simulink library "pmm"  (R2021b)
settings: Solver=VariableStepAuto  StartTime=0.0  StopTime=10.0  RelTol=1e-3
undefined symbols (not defined in the file or in its folder): APMM_CoolgFanActCurr_X_pct, APMM_EWP1Curr_X_c, APMM_EWP3Curr_X_c, APMM_LVBattChktime_X_enum, APMM_LVBattChrgtime_X_enum, APMM_LVChrgLv_X_mV, ENUM_ANTITHEFT_ALARM, ENUM_ANTITHEFT_ARM, ENUM_ANTITHEFT_DISARM, ENUM_ANTITHEFT_WAIT, ENUM_CHRGPLUGSTA_NONE, ENUM_CRASHSTATE_NOCRASH, ENUM_DCDCFAULTSTA_ANYFAULTLV1, ENUM_DCDCFAULTSTA_ANYFAULTLV2, ENUM_DRIVETRAIN_AWD, ENUM_DRIVETRAIN_FWD, ENUM_DRIVETRAIN_RWD, ENUM_GEARACTUALPOSN_D, ENUM_GEARACTUALPOSN_N, ENUM_GEARACTUALPOSN_R, ENUM_HVBATTREADYPRE_READY, ENUM_OTACHKSTA_NOREQUEST, ENUM_OTACHKSTA_NOTIMEOUT, ENUM_OTACHKSTA_TIMEOUT, ENUM_PDKEYRAWLULOCK_INLOCK, ENUM_PDKEYRAWLULOCK_INUNLOCK, ENUM_PDKEYRAWPS_INPS, ENUM_PDKEYSTA_LOCK, ENUM_PDKEYSTA_PS, ENUM_PDKEYSTA_UNAVALIABLE, ENUM_PDKEYSTA_UNLOCK, ENUM_POWERSTA_OFF, ENUM_POWERSTA_OFFC, ENUM_POWERSTA_STANDBY, ENUM_PWRREQOTA_REQPOWEROFF, ENUM_PWRREQOTA_REQPOWERSTDBY, ENUM_PWRSTASW_READY, FALSE, KPMM_AllDoorClosedHoldTime_s, KPMM_APSAllowThd_pct, KPMM_BattDownFailtime_s, KPMM_BattUpFailtime_s, KPMM_BattUpResetRty_cnt, KPMM_BattUpResetSW_flg, KPMM_BattUpResetTO_s, KPMM_BattUpRstDlyTO_s, KPMM_BrakeSWHoldTime_s, KPMM_ChrgPlugHoldTime_s, KPMM_DCDCDisableFailtime_s, KPMM_DCDCEnableFailtime_s, KPMM_DCDCVSET_V, KPMM_DCDCVSETLVChrg_V, KPMM_DoorSWHoldTime_s, KPMM_DriverSafetyChkFailtime_s, KPMM_DrivetrainSelect_enum_ovrdflg, KPMM_DrivetrainSelect_enum_ovrdval, KPMM_FDADC12VDetAccu_s, KPMM_FDADC12VDetAccuIntval_s, KPMM_FirstLVCheckHoldT_s, KPMM_FrMCUDischrgVolt_V ... (+54)
libraries: simulink x28, hcu_lib x13
(part 2 of 5)

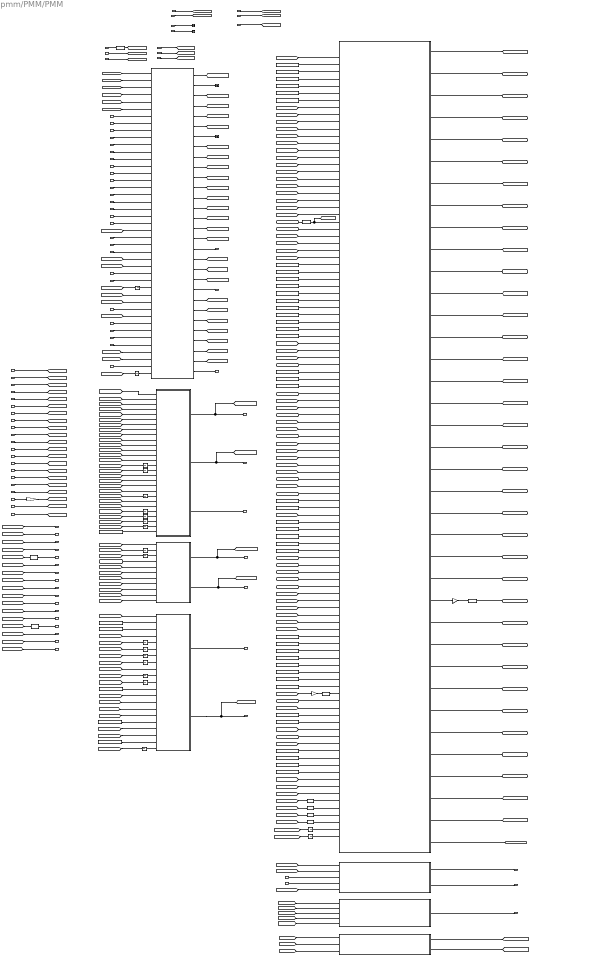
== system pmm/PMM/PMM ==
  note: VPMM_FirstFDADC12VDetAvg_mV
  note: BMS
  note: PEU
  note: 0 = open; 1 = close
  task_time_s : Inport
  VINP_DrDoorSW_flg : Inport  Port=2
  VINP_PsDoorSW_flg : Inport  Port=3
  VINP_RRDoorSW_flg : Inport  Port=4
  VINP_RLDoorSW_flg : Inport  Port=5
  VINP_BrakeSWGPIO_flg : Inport  Port=6
  VINP_SeatSW_flg : Inport  Port=7
  VINP_HoodSW_flg : Inport  Port=8
  VINP_TailgateSW_flg : Inport  Port=9
  VINP_CrashOutputSts_enum : Inport  Port=10
  VINP_VehSpeed_kph : Inport  Port=11
  VINP_IVIPwroffreq_flg : Inport  Port=12
  VINP_IVITriggerreq_flg : Inport  Port=13
  VINP_OFFACMODE_enum : Inport  Port=14
  VINP_AVMOFFRecButt_flg : Inport  Port=15
  VINP_SchedChgwake_flg : Inport  Port=16
  VINP_SchedChgbutt_flg : Inport  Port=17
  VINP_PWCONTINUEUSE_flg : Inport  Port=18
  VINP_DCDCReady4Pre_flg : Inport  Port=19
  VINP_DCDCEnabled_flg : Inport  Port=20
  VINP_OBCEnabled_flg : Inport  Port=21
  VINP_OBCReady4Pre_flg : Inport  Port=22
  VINP_OBCFaultStatus_enum : Inport  Port=23
  VINP_DCDCAuxVolt_V : Inport  Port=24
  VINP_FrMCUDCBusVolt_V : Inport  Port=25
  VINP_FrMCUDischrgSta_flg : Inport  Port=26
  VINP_FrMCUEnaSta_flg : Inport  Port=27
  VINP_FrMCUErr_enum : Inport  Port=28
  VINP_FrMCUReady4Pre_flg : Inport  Port=29
  VINP_FrMCUReady_flg : Inport  Port=30
  VINP_FrMCUTemp_C : Inport  Port=31
  VINP_RrMCUDCBusVolt_V : Inport  Port=32
  VINP_RrMCUDischrgSta_flg : Inport  Port=33
  VINP_RrMCUEnaSta_flg : Inport  Port=34
  VINP_RrMCUErr_enum : Inport  Port=35
  VINP_RrMCUReady4Pre_flg : Inport  Port=36
  VINP_RrMCUReady_flg : Inport  Port=37
  VINP_RrMCUTemp_C : Inport  Port=38
  VINP_HVBattReady4Pre_enum : Inport  Port=39
  VINP_ChrgPlugSta_enum : Inport  Port=40
  VINP_BMSREADY_flg : Inport  Port=41
  VINP_HVILSta_flg : Inport  Port=42
  VINP_HVBContactorSta_flg : Inport  Port=43
  VINP_ExtChrgSta_enum : Inport  Port=44
  VINP_HVBattSOC_pct : Inport  Port=45
  VINP_RrTMSpd_rpm : Inport  Port=46
  VINP_FrTMSpd_rpm : Inport  Port=47
  VINP_OBCPluginSta_flg : Inport  Port=48
  VINP_BMSWarn5_flg : Inport  Port=49
  VINP_BMSWarn6_flg : Inport  Port=50
  VINP_BMSWarn7_flg : Inport  Port=51
  VINP_BMSWarn8_flg : Inport  Port=52
  VINP_HVBPreheatPrecoolSta_enum : Inport  Port=53
  VINP_DCDCFaultSta_enum : Inport  Port=54
  VINP_CANMsgValidBMS2_flg : Inport  Port=55
  VINP_CANMsgValidBMS3_flg : Inport  Port=56
  VINP_FrEDURealTMTq_Nm : Inport  Port=57
  VINP_RrEDURealTMTq_Nm : Inport  Port=58
  VINP_DCDCAuxCur_A : Inport  Port=59
  VINP_V2LSta_enum : Inport  Port=60
  VINP_LVBattDet12V_V : Inport  Port=61
  VINP_PDKeyAreaPS_flg : Inport  Port=62
  VINP_PDKeyAreaLockUnlock_flg : Inport  Port=63
  VINP_PowerOffTSet_cnt : Inport  Port=64
  VINP_RePwrReqTbox_enum : Inport  Port=65
  VTQD_GearActualPosn_enum : Inport  Port=66
  VTQD_PBWLockTO_flg : Inport  Port=67
  VBCM_AntitheftSta_enum : Inport  Port=68
  VINP_AllowMovThd_OTA_enum : Inport  Port=69
  VINP_PwrReq_OTA_enum : Inport  Port=70
  VINP_DrivetrainSelect_enum : Inport  Port=71
  VINP_EvccAplusPwrUpReq_flg : Inport  Port=72
  VDHP_ActAPSPosn_pct : Inport  Port=73
  VDHP_EAPS12RangeSta_enum : Inport  Port=74
  VINP_FDEWP1Cmd_enum : Inport  Port=75
  VINP_FDEWP3Cmd_enum : Inport  Port=76
  VINP_CoolgFanActDuty_pct : Inport  Port=77
  VINP_PowerOffTSetDKC_enum : Inport  Port=78
  VINP_RePwrReqDKCT_enum : Inport  Port=79
  Constant : Constant  Value=KPMM_LVBattChkOKStdT_s
  Constant1 : Constant  Value=KPMM_LVBattThd_V
  Constant10 : Constant  Value=KPMM_OBCDisableFailtime_s
  Constant11 : Constant  Value=KPMM_DriverSafetyChkFailtime_s
  Constant12 : Constant  Value=KPMM_FDADC12VDetAccu_s
  Constant13 : Constant  Value=KPMM_PrechrgChkFailtime_s
  Constant14 : Constant  Value=KPMM_FirstLVCheckHoldT_s
  Constant15 : Constant  Value=KPMM_MLvSafetyFailtime_s
  Constant16 : Constant  Value=KPMM_MCUDisChrgFailtime_s
  Constant17 : Constant  Value=KPMM_DCDCVSET_V
  Constant18 : Constant  Value=KPMM_OFFStaByPassLVBatt_flg
  Constant19 : Constant  Value=KPMM_SilentChrgReq_flg_ovrdflg
  Constant2 : Constant  Value=KPMM_PwrStaStdTO_s
  Constant20 : Constant  Value=KPMM_DCDCEnableFailtime_s
  Constant21 : Constant  Value=KPMM_BattDownFailtime_s
  Constant22 : Constant  Value=KPMM_MCUDisableFailtime_s
  Constant23 : Constant  Value=KPMM_APSAllowThd_pct
  Constant24 : Constant  Value=KPMM_DCDCDisableFailtime_s
  Constant25 : Constant  Value=KPMM_SilentChrgReq_flg_ovrdval
  Constant27 : Constant  Value=KPMM_HVSOCWarnThd_pct
  Constant28 : Constant  Value=KPMM_HVBattSOCPwrDwnThd_pct
  Constant29 : Constant  Value=KPMM_HVSOCWarnThd_pct
  Constant3 : Constant  Value=KPMM_HVBattSOCThd_pct
  Constant30 : Constant  Value=KPMM_OffA2OffTime_s
  Constant31 : Constant  Value=KPMM_PluginVehSpdThd_kph
  Constant32 : Constant  Value=KPMM_LVChrgCurrMthd_flg
  Constant33 : Constant  Value=KPMM_LVChrgHoldT_s
  Constant34 : Constant  Value=KPMM_SysBaseCurr_A
  Constant35 : Constant  Value=KPMM_HVSOCWarnTime_s
  Constant36 : Constant  Value=KPMM_SilentChrgReqTO_s
  Constant37 : Constant  Value=KPMM_PwrStaONTOPop_s
  Constant38 : Constant  Value=KPMM_LVBattChkWakehold_s
  Constant39 : Constant  Value=KPMM_LVBattOFFSlpThd_mV
  Constant4 : Constant  Value=KPMM_HVBSOCOffStaChkFailtime_s
  Constant40 : Constant  Value=KPMM_OFFLVBattChkRetry_cnt
  Constant41 : Constant  Value=KPMM_SysPwrDownDbns_s
  Constant42 : Constant  Value=KPMM_BattUpResetRty_cnt
  Constant43 : Constant  Value=KPMM_BattUpResetSW_flg
  Constant44 : Constant  Value=KPMM_BattUpResetTO_s
  Constant45 : Constant  Value=KPMM_BattUpRstDlyTO_s
  Constant46 : Constant  Value=KPMM_HoodOffChkFailtime_s
  Constant47 : Constant  Value=KPMM_HVBattSOCPwrDwnThd_pct
  Constant5 : Constant  Value=KPMM_HVBSOCOFFCStaChkFailtime_s
  Constant6 : Constant  Value=KPMM_FDADC12VDetAccuIntval_s
  Constant7 : Constant  Value=KPMM_OBCPreChgChkFailtime_s
  Constant8 : Constant  Value=KPMM_SafetyChkFailtime_s
  Constant9 : Constant  Value=KPMM_BattUpFailtime_s  OutDataTypeStr=single
  DCDC output volt setpoint judgment : Subsystem
  Data Type Conversion : DataTypeConversion
  Data Type Conversion1 : DataTypeConversion
  Data Type Conversion2 : DataTypeConversion  OutDataTypeStr=single
  Data Type Conversion3 : DataTypeConversion  OutDataTypeStr=uint8
  Data Type Conversion39 : DataTypeConversion
  Data Type Conversion4 : DataTypeConversion  OutDataTypeStr=single
  Detect Decrease : simulink/Logic and Bit Operations/Detect Decrease  vinit=0.0  OutDataTypeStr=boolean
  Detect Increase : simulink/Logic and Bit Operations/Detect Increase  vinit=0.0  OutDataTypeStr=boolean
  Detect Increase1 : simulink/Logic and Bit Operations/Detect Increase  vinit=0.0  OutDataTypeStr=boolean
  Detect Increase2 : simulink/Logic and Bit Operations/Detect Increase  vinit=0.0  OutDataTypeStr=boolean
  Gain : Gain  Gain=MIN2SEC
  Gain1 : Gain  Gain=1000
  Gain2 : Gain  Gain=0.001
  MCU_EnaReq_Control : Subsystem
  OTA power state constrain : Subsystem
  PMMDataConvert : Subsystem  AncestorBlock=pmm/PMM/PowerModeManagement/PMMDataConvert
  PMM_State_Machine : Stateflow chart  TreatAsAtomicUnit=on
      settings: PortSchema="{\"entries\":[{\"content\":{\"sides\":[{\"content\":{\"connectorIds\":[\"In1\",\"In2\",\"In3\",\"In4\",\"In5\",\"In6\",\"In7\",\"In8\",\"In9\",\"In10\",\"In11\",\"In12\",\"In13\",\"In14\",\"In15\",\"In16\",\"In17\",\"In18\",\"In19\",\"In20\",\"In21\",\"In22\",\"In23\",\"In24\",\"In25\",\"In26\",\"In27\",\"In28\",\"In29\",\"In30\",\"In31\",\"In32\",\"In33\",\"In34\",\"In35\",\"In36\",\"In37\",\"In38\",\"In39\",\"In40\",\"In41\",\"In42\",\"In43\",\"In44\",\"In45\",\"In46\",\"In47\",\"In48\",\"In49\",\"In50\",\"In51\",\"In53\",\"In54\",\"In55\",\"In56\",\"In57\",\"In58\",\"In59\",\"In52\",\"In60\",\"In61\",\"In62\",\"In63\",\"In64\",\"In66\",\"In67\",\"In68\",\"In69\",\"In70\",\"In71\",\"In74\",\"In75\",\"In72\",\"In73\",\"In65\",\"In76\",\"In77\",\"In78\",\"In79\",\"In80\",\"In81\",\"In82\",\"In83\",\"In84\",\"In85\",\"In86\",\"In87\",\"In88\",\"In89\",\"In90\",\"In91\",\"In97\",\"In98\",\"In99\",\"In100\",\"In101\",\"In96\",\"In92\",\"In93\",\"In94\",\"In95\",\"In102\",\"In103\",\"In104\",\"In105\",\"In106\",\"In107\",\"In108\",\"In109\",\"In110\"]},\"type\":\"ConnectorPlacement.EquallySpacedRectSide\",\"uuid\":\"8ab1b0ff-73ed-4b41-8f3f-fcf16c31188d\"},{\"content\":{\"connectorIds\":[\"Out1\",\"Out2\",\"Out3\",\"Out4\",\"Out5\",\"Out6\",\"Out7\",\"Out8\",\"Out9\",\"Out10\",\"Out11\",\"Out12\",\"Out13\",\"Out14\",\"Out17\",\"Out18\",\"Out19\",\"Out20\",\"Out21\",\"Out22\",\"Out23\",\"Out24\",\"Out25\",\"Out26\",\"Out27\",\"Out28\",\"Out29\",\"Out30\",\"Out31\",\"Out32\",\"Out33\",\"Out34\",\"Out35\",\"Out36\",\"Out15\",\"Out16\",\"Out37\"],\"side\":\"RIGHT\"},\"type\":\"ConnectorPlacement.EquallySpacedRectSide\",\"uuid\":\"e75ad163-33ee-46d6-b33a-670f57cb3f5e\"},{\"content\":{\"connectorIds\":[],\"side\":\"TOP\"},\"type\":\"ConnectorPlacement.EquallySpacedRectSide\",\"uuid\":\"84c68278-d5af-48d1-859e-0f05090acbaa\"}]},\"type\":\"ConnectorPlacement.EquallySpacedConnector\",\"uuid\":\"278d3476-0e07-485b-a357-39a0667eafe4\"}],\"packageUris\":[\"http://schema.mathworks.com/mf0/Connector/R2020b\"],\"version\":\"1.0\"}"
  RequirementManagementForPowerDown : Stateflow chart  TreatAsAtomicUnit=on
  RequirementManagementForPowerStateConstrain : Stateflow chart  TreatAsAtomicUnit=on
      settings: PortSchema="{\"entries\":[{\"content\":{\"sides\":[{\"content\":{\"connectorIds\":[\"In1\",\"In2\",\"In11\",\"In3\",\"In4\",\"In5\",\"In6\",\"In7\",\"In8\",\"In9\",\"In10\"]},\"type\":\"ConnectorPlacement.EquallySpacedRectSide\",\"uuid\":\"c4039c9e-34d9-4d76-8a20-7739646b6da6\"},{\"content\":{\"connectorIds\":[\"Out1\",\"Out2\"],\"side\":\"RIGHT\"},\"type\":\"ConnectorPlacement.EquallySpacedRectSide\",\"uuid\":\"63e3e661-9024-478e-a9c0-8e66b2c0118c\"},{\"content\":{\"connectorIds\":[],\"side\":\"TOP\"},\"type\":\"ConnectorPlacement.EquallySpacedRectSide\",\"uuid\":\"6c94eba6-19b8-417a-9a11-c61323531ba8\"}]},\"type\":\"ConnectorPlacement.EquallySpacedConnector\",\"uuid\":\"e4d90d6b-0647-4724-8d20-4a3edeab4c97\"}],\"packageUris\":[\"http://schema.mathworks.com/mf0/Connector/R2020b\"],\"version\":\"1.0\"}"
  RequirementManagementForPowerUp : Stateflow chart  TreatAsAtomicUnit=on
  Terminator{,1..3} (4 alike) : Terminator
  Unit Delay{,1..19} (20 alike) : UnitDelay  SampleTime=-1  HasFrameUpgradeWarning=on
  VPMM_PowerUpState_enum : Outport
  VPMM_PowerDownState_enum : Outport  Port=2
  VPMM_PowerUpFault_enum : Outport  Port=3
  VPMM_PowerDownFault_enum : Outport  Port=4
  VPMM_ActiveDischargeReq_flg : Outport  Port=5
  VPMM_DCDCEnaReq_flg : Outport  Port=6
  VPMM_DCDCVoltSetpoint_V : Outport  Port=7
  VPMM_HVBatCnctReq_flg : Outport  Port=8
  VPMM_HVSysReadyToCharge_enum : Outport  Port=9
  VPMM_PowerSta_enum : Outport  Port=10
  VPMM_LVPwrSta_flg : Outport  Port=11
  VPMM_HVPwrSta_flg : Outport  Port=12
  VPMM_SysPowerMode_enum : Outport  Port=13
  VPMM_FrMCUEnaReq_flg : Outport  Port=14
  VPMM_RrMCUEnaReq_flg : Outport  Port=15
  VPMM_DrivetrainSelect_enum : Outport  Port=16
  VPMM_DrSeatSta_enum : Outport  Port=17
  VPMM_PwrStaSelect_enum : Outport  Port=18
  VPMM_PwrStaConstraint_enum : Outport  Port=19
  VPMM_TCountSta_enum : Outport  Port=20
  VPMM_PwrUpReq_enum : Outport  Port=21
  VPMM_PwrDownReq_enum : Outport  Port=22
  VPMM_LowSOCWarn_enum : Outport  Port=23
  VPMM_ReVehThdChkSta_enum : Outport  Port=24
  VPMM_LVSysErrPwrOutErr_flg : Outport  Port=25
  VPMM_EvccAplusPwrUpReq_flg : Outport  Port=26
  VPMM_PwrStaONTOPopReq_flg : Outport  Port=27
  VPMM_IVIPwrStaONTOPopT_s : Outport  Port=28
  VPMM_LVChrgHoldTtimer_s : Outport  Port=29
  VPMM_LVBattChrgTimeCnt_s : Outport  Port=30
  VPMM_SilentChkAllowSleep_flg : Outport  Port=31
  VPMM_TimerAllowSleep_flg : Outport  Port=32
  VPMM_FDADC12VDetAvg_mV : Outport  Port=33
  VPMM_PMMAllowECUSleep_flg : Outport  Port=34
  VPMM_LVSilentChrgSta_enum : Outport  Port=35
  VPMM_LVSilentChrgReq_flg : Outport  Port=36
  VPMM_LVSilentChrgLv_enum : Outport  Port=37
  VPMM_LVBattChktime_s : Outport  Port=38
  VPMM_SafetyChkMLv_flg : Outport  Port=39
  VPMM_SafetyChkHLv_flg : Outport  Port=40
  VPMM_HVChrgPreActionErrSta_enum : Outport  Port=41
  VPMM_MCUReady_flg : Outport  Port=42
  VPMM_MCUReady4Pre_flg : Outport  Port=43
  VPMM_CtrlFrPwrStbA1P_flg : Outport  Port=44
  VPMM_CtrlFrRC1_flg : Outport  Port=45
  VPMM_CtrlFrBMSCCUCIR_flg : Outport  Port=46
  VPMM_CtrlFrEDUINVERTER_flg : Outport  Port=47
  VPMM_HWResetSta_enum : Outport  Port=48
  VPMM_CtrlDrPwrStbA2_flg : Outport  Port=49
  VPMM_PwrStaTOSta_enum : Outport  Port=50
  VPMM_PMMAllowNMSleep_flg : Outport  Port=51
  VPMM_Sched_ChgTOSta_enum : Outport  Port=52
  VPMM_PwrReq_OTA_enum : Outport  Port=53
  VPMM_OTAPwrReqOFFChkSta_enum : Outport  Port=54
  VPMM_OTAPwrReqStdChkSta_enum : Outport  Port=55
  VPMM_MCUDCBusMaxVolt_V : Outport  Port=56
  wires:
  PMM_State_Machine/16(VPMM_PwrStaTOSta_enum) -> [VPMM_PwrStaTOSta_enum]  "VPMM_PwrStaTOSta_enum"
  PMM_State_Machine/17(VPMM_Sched_ChgTOSta_enum) -> [VPMM_Sched_ChgTOSta_enum]  "VPMM_Sched_ChgTOSta_enum"
  PMM_State_Machine/15(VPMM_LVSilentChrgReq_flg) -> [VPMM_LVSilentChrgReq_flg]  "VPMM_LVSilentChrgReq_flg"
  PMM_State_Machine/18(VPMM_LVSilentChrgReqStd_flg) -> [VPMM_LVSilentChrgReqStd_flg]  "VPMM_LVSilentChrgReqStd_flg"
  VDHP_EAPS12RangeSta_enum/1 -> PMM_State_Machine/65(VDHP_EAPS12RangeSta_enum)
  Constant2/1 -> PMM_State_Machine/64(KPMM_PwrStaStdTO_s)
  Constant/1 -> PMM_State_Machine/63(KPMM_LVBattChkOKStdT_s)
  [VINP_EvccAplusPwrUpReq_flg] -> RequirementManagementForPowerUp/23(VINP_EvccAplusPwrUpReq_flg)
  VINP_EvccAplusPwrUpReq_flg/1 -> [VINP_EvccAplusPwrUpReq_flg]
  [VPMM_LVSilentChrgReqStd_flg] -> Unit Delay8/1
  Unit Delay8/1 -> RequirementManagementForPowerUp/24(VPMM_LVSilentChrgReqStd_flg)
  [VINP_ChrgPlugSta_enum] -> RequirementManagementForPowerUp/22(VINP_ChrgPlugSta_enum)
  [VINP_PwrReq_OTA_enum] -> PMM_State_Machine/61(VINP_PwrReq_OTA_enum)
  Unit Delay7/1 -> RequirementManagementForPowerDown/10(VPMM_Sched_ChgTOSta_enum)
  [VPMM_Sched_ChgTOSta_enum] -> Unit Delay7/1
  [VPMM_PowerUpState_enum] -> Unit Delay1/1
  Unit Delay1/1 -> RequirementManagementForPowerUp/21(VPMM_PowerUpState_enum)
  [task_time_s] -> RequirementManagementForPowerUp/1(task_time_s)
  [VPMM_DrivetrainSelect_enum] -> MCU_EnaReq_Control/5(VPMM_DrivetrainSelect_enum)
  MCU_EnaReq_Control/2(VPMM_RrMCUEnaReq_flg) -> VPMM_RrMCUEnaReq_flg/1  "VPMM_RrMCUEnaReq_flg"
  MCU_EnaReq_Control/1(VPMM_FrMCUEnaReq_flg) -> VPMM_FrMCUEnaReq_flg/1  "VPMM_FrMCUEnaReq_flg"
  Unit Delay6/1 -> PMMDataConvert/31(VPMM_PowerSta_enum)
  Unit Delay5/1 -> RequirementManagementForPowerDown/5(VPMM_PowerSta_enum)
  Unit Delay4/1 -> RequirementManagementForPowerStateConstrain/2(VPMM_PowerSta_enum)
  Unit Delay3/1 -> RequirementManagementForPowerUp/15(VPMM_LVSilentChrgReq_flg)
  [VPMM_AllDoorClosed_flg] -> RequirementManagementForPowerUp/8(VPMM_AllDoorClosed_flg)
  Unit Delay2/1 -> RequirementManagementForPowerDown/7(VPMM_PwrStaTOSta_enum)
  Unit Delay/1 -> RequirementManagementForPowerUp/16(VPMM_PowerSta_enum)
  VINP_CANMsgValidBMS3_flg/1 -> PMM_State_Machine/60(VINP_CANMsgValidBMS3_flg)
  PMM_State_Machine/14(VPMM_LVBattChktime_s) -> VPMM_LVBattChktime_s/1  "VPMM_LVBattChktime_s"
  [VPMM_PwrUpReq_enum] -> PMM_State_Machine/59(VPMM_PwrUpReq_enum)
  [VPMM_PwrStaSelect_enum] -> PMM_State_Machine/58(VPMM_PwrStaSelect_enum)
  [VPMM_PwrStaConstraint_enum] -> PMM_State_Machine/57(VPMM_PwrStaConstraint_enum)
  [VPMM_PwrDownReq_enum] -> PMM_State_Machine/56(VPMM_PwrDownReq_enum)
  VINP_AllowMovThd_OTA_enum/1 -> PMM_State_Machine/55(VINP_AllowMovThd_OTA_enum)
  [VINP_RePwrReqTbox_enum] -> RequirementManagementForPowerDown/9(VINP_RePwrReqTbox_enum)
  [VPMM_TCountSta_enum] -> Unit Delay12/1
  [VPMM_PwrStaTOSta_enum] -> Unit Delay2/1
  [VINP_HVBattSOC_pct] -> RequirementManagementForPowerDown/4(VINP_HVBattSOC_pct)
  [VINP_RePwrReqTbox_enum] -> RequirementManagementForPowerUp/20(VINP_RePwrReqTbox_enum)
  [VINP_RePwrReqDKCT_enum] -> RequirementManagementForPowerUp/19(VINP_RePwrReqDKCT_enum)
  VINP_PowerOffTSetDKC_enum/1 -> [VINP_PowerOffTSetDKC_enum]
  VINP_RePwrReqDKCT_enum/1 -> [VINP_RePwrReqDKCT_enum]
  VINP_RePwrReqTbox_enum/1 -> [VINP_RePwrReqTbox_enum]
  [VINP_PwrReq_OTA_enum] -> RequirementManagementForPowerUp/18(VINP_PwrReq_OTA_enum)
  VINP_PwrReq_OTA_enum/1 -> [VINP_PwrReq_OTA_enum]
  [VTQD_GearActualPosn_enum] -> RequirementManagementForPowerUp/17(VTQD_GearActualPosn_enum)
  [VTQD_GearActualPosn_enum] -> PMM_State_Machine/29(VTQD_GearActualPosn_enum)
  VTQD_GearActualPosn_enum/1 -> [VTQD_GearActualPosn_enum]
  [VPMM_DetectDoorOpened_flg] -> RequirementManagementForPowerUp/14(VPMM_DetectDoorOpened_flg)
  [VPMM_ChrgPlugInRisingEdge_flg] -> RequirementManagementForPowerUp/13(VPMM_ChrgPlugInRisingEdge_flg)
  [VPMM_LVSilentChrgReq_flg] -> Unit Delay3/1
  [VPMM_BrkPedalRisingEdge_flg] -> RequirementManagementForPowerUp/12(VPMM_BrkPedalRisingEdge_flg)
  [VBCM_AntitheftSta_enum] -> RequirementManagementForPowerUp/9(VBCM_AntitheftSta_enum)
  [VINP_HVBattSOC_pct] -> RequirementManagementForPowerUp/3(VINP_HVBattSOC_pct)
  [VINP_HVBattSOC_pct] -> PMM_State_Machine/28(VINP_HVBattSOC_pct)
  VINP_HVBattSOC_pct/1 -> [VINP_HVBattSOC_pct]
  VINP_SchedChgbutt_flg/1 -> PMM_State_Machine/51(VINP_SchedChgbutt_flg)
  [VINP_TailgateSW_flg] -> RequirementManagementForPowerUp/5(VINP_TailgateSW_flg)
  [VINP_HoodSW_flg] -> RequirementManagementForPowerUp/4(VINP_HoodSW_flg)
  [VINP_HoodSW_flg] -> PMM_State_Machine/54(VINP_HoodSW_flg)
  VINP_TailgateSW_flg/1 -> [VINP_TailgateSW_flg]
  VINP_HoodSW_flg/1 -> [VINP_HoodSW_flg]
  [VINP_HVBPreheatPrecoolSta_enum] -> RequirementManagementForPowerUp/2(VINP_HVBPreheatPrecoolSta_enum)
  VINP_HVBPreheatPrecoolSta_enum/1 -> [VINP_HVBPreheatPrecoolSta_enum]
  [VPMM_PwrStaConstraint_enum] -> Unit Delay11/1
  [VPMM_BrkPedalPressed_flg] -> RequirementManagementForPowerUp/11(VPMM_BrkPedalPressed_flg)
  [VPMM_BMSWarm_flg] -> RequirementManagementForPowerUp/10(VPMM_BMSWarn_flg)
  [VPMM_PowerSta_enum] -> Unit Delay/1
  [VPMM_PowerSta_enum] -> Unit Delay5/1
  [VPMM_PowerSta_enum] -> Unit Delay4/1
  [task_time_s] -> RequirementManagementForPowerDown/1(task_time_s)
  [task_time_s] -> RequirementManagementForPowerStateConstrain/1(task_time_s)
  Constant30/1 -> RequirementManagementForPowerDown/3(KPMM_OffA2OffTime_s)
  Constant29/1 -> RequirementManagementForPowerDown/2(KPMM_HVSOCWarnThd_pct)
  [VBCM_AntitheftSta_enum] -> PMMDataConvert/2(VBCM_AntitheftSta_enum)
  VBCM_AntitheftSta_enum/1 -> [VBCM_AntitheftSta_enum]
  [VPMM_MCUDCBusMaxVolt_V] -> PMM_State_Machine/52(VPMM_MCUDCBusMaxVolt_V)
  [VINP_DrDoorSW_flg] -> PMM_State_Machine/53(VINP_DrDoorSW_flg)
  [VPMM_SeatSWRisingEdge_flg] -> PMM_State_Machine/50(VPMM_SeatSWRisingEdge_flg)
  [VPMM_ChrgPlugOutFallingEdge_flg] -> PMM_State_Machine/49(VPMM_ChrgPlugFallingEdge_flg)
  VINP_OBCPluginSta_flg/1 -> PMM_State_Machine/48(VINP_OBCPluginSta_flg)
  Constant18/1 -> PMM_State_Machine/47(KPMM_OFFStaByPassLVBatt_flg)
  Constant25/1 -> PMM_State_Machine/46(KPMM_SilentChrgReq_flg_ovrdval)
  Constant19/1 -> PMM_State_Machine/45(KPMM_SilentChrgReq_flg_ovrdflg)
  VTQD_PBWLockTO_flg/1 -> PMM_State_Machine/44(VTQD_EnterPGearFail_flg)
  [VPMM_AllDoorCloseRisingEdge_flg] -> PMM_State_Machine/43(VPMM_AllDoorCloseRisingEdge_flg)
  [VINP_DCDCEnabled_flg] -> PMM_State_Machine/41(VINP_DCDCEnabled_flg)
  Constant17/1 -> PMM_State_Machine/40(KPMM_DCDCVSET_V)
  Constant16/1 -> PMM_State_Machine/39(KPMM_MCUDisChrgFailtime_s)
  Constant15/1 -> PMM_State_Machine/38(KPMM_MLvSafetyFailtime_s)
  [VPMM_PDKeySta_enum] -> PMM_State_Machine/26(VPMM_PDKeySta_enum)
  Constant13/1 -> PMM_State_Machine/37(KPMM_PrechrgChkFailtime_s)
  [VINP_SeatSW_flg] -> PMM_State_Machine/27(VINP_SeatSW_flg)
  Constant11/1 -> PMM_State_Machine/36(KPMM_DriverSafetyChkFailtime_s)
  Constant8/1 -> PMM_State_Machine/35(KPMM_SafetyChkFailtime_s)
  Constant7/1 -> PMM_State_Machine/34(KPMM_OBCPreChgChkFailtime_s)
  Constant1/1 -> PMM_State_Machine/30(KPMM_LVBattThd_V)
  Constant5/1 -> PMM_State_Machine/33(KPMM_HVBSOCOFFCStaChkFailtime_s)
  Constant3/1 -> PMM_State_Machine/31(KPMM_HVBattSOCThd_pct)
  Constant4/1 -> PMM_State_Machine/32(KPMM_HVBSOCOffStaChkFailtime_s)
  VINP_IVITriggerreq_flg/1 -> PMM_State_Machine/25(VINP_IVITriggerreq_flg)
  [VPMM_SafetyChkMLv_flg] -> PMM_State_Machine/23(VPMM_SafetyChkMLv_flg)
  [VPMM_SafetyChkHLv_flg] -> PMM_State_Machine/22(VPMM_SafetyChkHLv_flg)
  [VINP_OBCEnabled_flg] -> PMM_State_Machine/21(VINP_OBCEnabled_flg)
  [VINP_OBCReady4Pre_flg] -> PMM_State_Machine/20(VINP_OBCReady4Pre_flg)
  [VPMM_BrkPedalRisingEdge_flg] -> PMM_State_Machine/19(VPMM_BrkPedalRisingEdge_flg)
  [VPMM_MCUReady_flg] -> PMM_State_Machine/18(VPMM_MCUReady_flg)
  [VPMM_BrkPedalPressed_flg] -> PMM_State_Machine/17(VPMM_BrkPedalPressed_flg)
  [VPMM_AllDoorClosed_flg] -> PMM_State_Machine/16(VPMM_AllDoorClosed_flg)
  [VPMM_PreChrgChk_flg] -> PMM_State_Machine/15(VPMM_PreChrgChk_flg)
  [VPMM_MCUEnable_flg] -> PMM_State_Machine/14(VPMM_MCUEnable_flg)
  [VPMM_DetectDoorOpened_flg] -> PMM_State_Machine/13(VPMM_DetectDoorOpened_flg)
  [VINP_HVBContactorSta_flg] -> PMM_State_Machine/12(VINP_HVBContactorSta_flg)
  [VINP_ChrgPlugSta_enum] -> PMM_State_Machine/11(VINP_ChrgPlugSta_enum)
  [VINP_ExtChrgSta_enum] -> PMM_State_Machine/9(VINP_ExtChrgSta_enum)
  [VINP_BMSREADY_flg] -> PMM_State_Machine/8(VINP_BMSREADY_flg)
  Constant10/1 -> PMM_State_Machine/7(KPMM_OBCDisableFailtime_s)
  Constant24/1 -> PMM_State_Machine/6(KPMM_DCDCDisableFailtime_s)
  Constant22/1 -> PMM_State_Machine/5(KPMM_MCUDisableFailtime_s)
  Constant21/1 -> PMM_State_Machine/4(KPMM_BattDownFailtime_s)
  Constant20/1 -> PMM_State_Machine/3(KPMM_DCDCEnableFailtime_s)
  Constant9/1 -> PMM_State_Machine/2(KPMM_BattUpFailtime_s)
  [task_time_s] -> PMM_State_Machine/1(task_time_s)
  RequirementManagementForPowerUp/3(VPMM_ReVehThdChkSta_enum) -> VPMM_ReVehThdChkSta_enum/1  "VPMM_ReVehThdChkSta_enum"
  RequirementManagementForPowerDown/1(VPMM_LowSOCWarn_enum) -> VPMM_LowSOCWarn_enum/1  "VPMM_LowSOCWarn_enum"
  RequirementManagementForPowerDown/2(VPMM_PwrDownReq_enum) -> [VPMM_PwrDownReq_enum], VPMM_PwrDownReq_enum/1  "VPMM_PwrDownReq_enum"
  RequirementManagementForPowerUp/2(VPMM_PwrUpReq_enum) -> VPMM_PwrUpReq_enum/1, [VPMM_PwrUpReq_enum]  "VPMM_PwrUpReq_enum"
  RequirementManagementForPowerStateConstrain/2(VPMM_TCountSta_enum) -> VPMM_TCountSta_enum/1, [VPMM_TCountSta_enum]  "VPMM_TCountSta_enum"
  RequirementManagementForPowerStateConstrain/1(VPMM_PwrStaConstraint_enum) -> VPMM_PwrStaConstraint_enum/1, [VPMM_PwrStaConstraint_enum]  "VPMM_PwrStaConstraint_enum"
  RequirementManagementForPowerUp/1(VPMM_PwrStaSelect_enum) -> VPMM_PwrStaSelect_enum/1, [VPMM_PwrStaSelect_enum]  "VPMM_PwrStaSelect_enum"
  PMMDataConvert/18(VPMM_DrSeatSta_enum) -> VPMM_DrSeatSta_enum/1
  [VINP_DrDoorSW_flg] -> PMMDataConvert/3(VINP_DrDoorSW_flg)
  VINP_DrDoorSW_flg/1 -> [VINP_DrDoorSW_flg]
  PMMDataConvert/20(VPMM_MCUDCBusMaxVolt_V) -> [VPMM_MCUDCBusMaxVolt_V]
  VINP_RrMCUErr_enum/1 -> PMMDataConvert/18(VINP_RrMCUErr_enum)
  VINP_RrMCUEnaSta_flg/1 -> PMMDataConvert/17(VINP_RrMCUEnaSta_flg)
  VINP_RrMCUDischrgSta_flg/1 -> PMMDataConvert/16(VINP_RrMCUDischrgSta_flg)
  VINP_RrMCUDCBusVolt_V/1 -> PMMDataConvert/15(VINP_RrMCUDCBusVolt_V)
  VINP_FrMCUTemp_C/1 -> PMMDataConvert/14(VINP_FrMCUTemp_C)
  VINP_FrMCUReady_flg/1 -> PMMDataConvert/13(VINP_FrMCUReady_flg)
  VINP_FrMCUReady4Pre_flg/1 -> PMMDataConvert/12(VINP_FrMCUReady4Pre_flg)
  VINP_FrMCUErr_enum/1 -> PMMDataConvert/11(VINP_FrMCUErr_enum)
  VINP_FrMCUEnaSta_flg/1 -> PMMDataConvert/10(VINP_FrMCUEnaSta_flg)
  VINP_FrMCUDischrgSta_flg/1 -> PMMDataConvert/9(VINP_FrMCUDischrgSta_flg)
  VINP_FrMCUDCBusVolt_V/1 -> PMMDataConvert/8(VINP_FrMCUDCBusVolt_V)
  VINP_BrakeSWGPIO_flg/1 -> PMMDataConvert/7(VINP_BrakeSWGPIO_flg)
  PMMDataConvert/19(VPMM_BMSWarm_flg) -> [VPMM_BMSWarm_flg]
  VINP_BMSWarn8_flg/1 -> PMMDataConvert/37(VINP_BMSWarn8_flg)
  VINP_BMSWarn7_flg/1 -> PMMDataConvert/36(VINP_BMSWarn7_flg)
  VINP_BMSWarn5_flg/1 -> PMMDataConvert/34(VINP_BMSWarn5_flg)
  [VINP_FrTMSpd_rpm] -> PMMDataConvert/33(VINP_FrTMSpd_rpm)
  [VINP_RrTMSpd_rpm] -> PMMDataConvert/32(VINP_RrTMSpd_rpm)
  VINP_FrTMSpd_rpm/1 -> [VINP_FrTMSpd_rpm]
  VINP_RrTMSpd_rpm/1 -> [VINP_RrTMSpd_rpm]
  PMMDataConvert/15(VPMM_SeatSWRisingEdge_flg) -> [VPMM_SeatSWRisingEdge_flg]
  PMMDataConvert/14(VPMM_ChrgPlugOutFallingEdge_flg) -> [VPMM_ChrgPlugOutFallingEdge_flg]
  PMMDataConvert/17(VPMM_SafetyChkHLv_flg) -> [VPMM_SafetyChkHLv_flg]
  PMMDataConvert/16(VPMM_SafetyChkMLv_flg) -> [VPMM_SafetyChkMLv_flg]
  PMMDataConvert/13(VPMM_ChrgPlugInRisingEdge_flg) -> [VPMM_ChrgPlugInRisingEdge_flg]
  [VINP_SeatSW_flg] -> PMMDataConvert/28(VINP_SeatSW_flg)
  VINP_SeatSW_flg/1 -> [VINP_SeatSW_flg]
  [VPMM_PowerSta_enum] -> Unit Delay6/1
  VINP_CrashOutputSts_enum/1 -> PMMDataConvert/30(VINP_CrashOutputSts_enum)
  VINP_HVILSta_flg/1 -> PMMDataConvert/29(VINP_HVILSta_flg)
  VINP_OBCFaultStatus_enum/1 -> Terminator/1
  [VPMM_DrivetrainSelect_enum] -> VPMM_DrivetrainSelect_enum/1  "VPMM_DrivetrainSelect_enum"
  PMMDataConvert/12(VPMM_DrivetrainSelect_enum) -> [VPMM_DrivetrainSelect_enum]
  PMMDataConvert/11(VPMM_AllDoorCloseRisingEdge_flg) -> [VPMM_AllDoorCloseRisingEdge_flg]
  VINP_HVBContactorSta_flg/1 -> [VINP_HVBContactorSta_flg]
  VINP_ExtChrgSta_enum/1 -> [VINP_ExtChrgSta_enum]
  VINP_DCDCAuxVolt_V/1 -> Terminator3/1
  task_time_s/1 -> Data Type Conversion4/1
  VINP_ChrgPlugSta_enum/1 -> [VINP_ChrgPlugSta_enum]
  VINP_OBCEnabled_flg/1 -> [VINP_OBCEnabled_flg]
  VINP_BMSREADY_flg/1 -> [VINP_BMSREADY_flg]
  VINP_DCDCEnabled_flg/1 -> [VINP_DCDCEnabled_flg]
  VINP_OBCReady4Pre_flg/1 -> [VINP_OBCReady4Pre_flg]
  VINP_HVBattReady4Pre_enum/1 -> PMMDataConvert/24(VINP_HVBattReady4Pre_enum)
  VINP_DCDCReady4Pre_flg/1 -> PMMDataConvert/22(VINP_DCDCReady4Pre_flg)
  VINP_RrMCUTemp_C/1 -> PMMDataConvert/21(VINP_RrMCUTemp_C)
  VINP_RrMCUReady_flg/1 -> PMMDataConvert/20(VINP_RrMCUReady_flg)
  PMM_State_Machine/12(VPMM_HVPwrSta_flg) -> [VPMM_HVPwrSta_flg]  "VPMM_HVPwrSta_flg"
  PMM_State_Machine/11(VPMM_LVPwrSta_flg) -> VPMM_LVPwrSta_flg/1  "VPMM_LVPwrSta_flg"
  PMM_State_Machine/8(VPMM_HVBatCnctReq_flg) -> VPMM_HVBatCnctReq_flg/1  "VPMM_HVBatCnctReq_flg"
  VINP_RrMCUReady4Pre_flg/1 -> PMMDataConvert/19(VINP_RrMCUReady4Pre_flg)
  PMM_State_Machine/6(VPMM_DCDCEnaReq_flg) -> VPMM_DCDCEnaReq_flg/1  "VPMM_DCDCEnaReq_flg"
  VINP_PDKeyAreaLockUnlock_flg/1 -> PMMDataConvert/26(VINP_PDKeyAreaLockUnlock_enum)
  PMMDataConvert/5(VPMM_AllDoorClosed_flg) -> [VPMM_AllDoorClosed_flg]
  PMMDataConvert/10(VPMM_BrkPedalRisingEdge_flg) -> [VPMM_BrkPedalRisingEdge_flg]
  PMMDataConvert/4(VPMM_PreChrgChk_flg) -> [VPMM_PreChrgChk_flg]
  PMM_State_Machine/9(VPMM_HVSysReadyToCharge_enum) -> VPMM_HVSysReadyToCharge_enum/1  "VPMM_HVSysReadyToCharge_enum"
  PMMDataConvert/1(VPMM_DetectDoorOpened_flg) -> [VPMM_DetectDoorOpened_flg]
  PMMDataConvert/2(VPMM_DetectDoorClosed_flg) -> Terminator1/1
  [task_time_s] -> PMMDataConvert/1(task_time_s)
  PMMDataConvert/3(VPMM_BrkPedalPressed_flg) -> [VPMM_BrkPedalPressed_flg]
  VINP_PDKeyAreaPS_flg/1 -> PMMDataConvert/25(VINP_PDKeyAreaPS_enum)
  PMMDataConvert/9(VPMM_PDKeySta_enum) -> [VPMM_PDKeySta_enum]
  PMM_State_Machine/10(VPMM_PowerSta_enum) -> [VPMM_PowerSta_enum]  "VPMM_PowerSta_enum"
  PMMDataConvert/8(VPMM_MCUReady_flg) -> [VPMM_MCUReady_flg]
  PMMDataConvert/6(VPMM_MCUEnable_flg) -> [VPMM_MCUEnable_flg]
  VINP_PowerOffTSet_cnt/1 -> Gain/1
  Gain/1 -> [VPMM_PowerOffTSet_s]  "VPMM_PowerOffTSet_s"
  VINP_DrivetrainSelect_enum/1 -> PMMDataConvert/38(VINP_DrivetrainSelect_enum)
  PMMDataConvert/21(VPMM_DetectAntitheftUnlock_flg) -> [VPMM_DetectAntitheftUnlock_flg]
  [VPMM_DetectAntitheftUnlock_flg] -> PMM_State_Machine/10(VPMM_DetectAntitheftUnlock_flg)
  PMM_State_Machine/19(VPMM_PreOFF_flg) -> [VPMM_PreOFF_flg]  "VPMM_PreOFF_flg"
  [VPMM_PreOFF_flg] -> Unit Delay10/1
  Unit Delay10/1 -> RequirementManagementForPowerUp/25(VPMM_PreOFF_flg)
  VDHP_ActAPSPosn_pct/1 -> PMM_State_Machine/62(VDHP_ActAPSPosn_pct)
  VINP_VehSpeed_kph/1 -> [VINP_VehSpeed_kph]
  [VINP_VehSpeed_kph] -> RequirementManagementForPowerUp/7(VINP_VehSpeed_kph)
  [VINP_VehSpeed_kph] -> PMM_State_Machine/66(VINP_VehSpeed_kph)
  Constant23/1 -> PMM_State_Machine/67(KPMM_APSAllowThd_pct)
  Constant31/1 -> PMM_State_Machine/68(KPMM_PluginVehSpdThd_kph)
  PMMDataConvert/7(VPMM_MCUDischrgFinished_flg) -> Terminator2/1
  VINP_DCDCFaultSta_enum/1 -> PMMDataConvert/39(VINP_DCDCFaultSta_enum)
  [VINP_ChrgPlugSta_enum] -> PMMDataConvert/27(VINP_ChrgPlugSta_enum)
  [VINP_OBCReady4Pre_flg] -> PMMDataConvert/23(VINP_OBCReady4Pre_flg)
  PMMDataConvert/22(VPMM_LVSysErrPwrOutErr_flg) -> VPMM_LVSysErrPwrOutErr_flg/1
  PMM_State_Machine/13(VPMM_PwrStaSW_enum) -> [VPMM_SysPowerMode_enum]  "VPMM_SysPowerMode_enum"
  [VPMM_SysPowerMode_enum] -> VPMM_SysPowerMode_enum/1
  [VPMM_PowerSta_enum] -> VPMM_PowerSta_enum/1
  [VPMM_PowerUpState_enum] -> VPMM_PowerUpState_enum/1
  [VPMM_SysPowerMode_enum] -> MCU_EnaReq_Control/1(VPMM_SysPowerMode_enum)
  VINP_FrEDURealTMTq_Nm/1 -> MCU_EnaReq_Control/3(VINP_FrEDURealTMTq_Nm)
  VINP_RrEDURealTMTq_Nm/1 -> MCU_EnaReq_Control/4(VINP_RrEDURealTMTq_Nm)
  [VTQD_GearActualPosn_enum] -> MCU_EnaReq_Control/2(VTQD_GearActualPosn_enum)
  VINP_DCDCAuxCur_A/1 -> PMM_State_Machine/73(VINP_DCDCAuxCur_A)
  Constant33/1 -> PMM_State_Machine/70(KPMM_LVChrgHoldT_s)
  Constant34/1 -> PMM_State_Machine/71(KPMM_SysBaseCurr_A)
  Constant32/1 -> PMM_State_Machine/69(KPMM_LVChrgCurrMthd_flg)
  VINP_FDEWP1Cmd_enum/1 -> PMM_State_Machine/74(VINP_FDEWP1Cmd_enum)
  VINP_FDEWP3Cmd_enum/1 -> PMM_State_Machine/75(VINP_FDEWP3Cmd_enum)
  VINP_CoolgFanActDuty_pct/1 -> PMM_State_Machine/72(VINP_CoolgFanActDuty_pct)
  PMM_State_Machine/20(VPMM_LVSilentChrgSta_enum) -> [VPMM_LVSilentChrgSta_enum]  "VPMM_LVSilentChrgSta_enum"
  [VPMM_LVSilentChrgSta_enum] -> Unit Delay9/1
  Unit Delay9/1 -> RequirementManagementForPowerDown/11(VPMM_LVSilentChrgSta_enum)
  PMMDataConvert/23(VPMM_DetectPDKeyUnlock_flg) -> [VPMM_DetectPDKeyUnlock_flg]
  [VPMM_DetectPDKeyUnlock_flg] -> PMM_State_Machine/76(VPMM_DetectPDKeyUnlock_flg)
  PMMDataConvert/24(VPMM_DetectAntitheftLock_flg) -> [VPMM_DetectAntitheftLock_flg]
  [VPMM_DetectAntitheftLock_flg] -> PMM_State_Machine/77(VPMM_DetectAntitheftLock_flg)
  PMMDataConvert/25(VPMM_DetectPDKeyLock_flg) -> [VPMM_DetectPDKeyLock_flg]
  [VPMM_DetectPDKeyLock_flg] -> PMM_State_Machine/78(VPMM_DetectPDKeyLock_flg)
  VINP_IVIPwroffreq_flg/1 -> [VINP_IVIPwroffreq_flg]
  [VINP_IVIPwroffreq_flg] -> PMM_State_Machine/42(VINP_IVIPwroffreq_flg)
  VINP_SchedChgwake_flg/1 -> [VINP_SchedChgwake_flg]
  [VINP_SchedChgwake_flg] -> RequirementManagementForPowerUp/6(VINP_SchedChgwake_flg)
  [VINP_IVIPwroffreq_flg] -> PMMDataConvert/40(VINP_IVIPwroffreq_flg)
  [VINP_SchedChgwake_flg] -> PMMDataConvert/41(VINP_SchedChgwake_flg)
  PMMDataConvert/26(VPMM_DetectIVIPwroffreq_flg) -> [VPMM_DetectIVIPwroffreq_flg]
  PMMDataConvert/27(VPMM_DetectSchedChg_flg) -> [VPMM_DetectSchedChg_flg]
  VINP_PWCONTINUEUSE_flg/1 -> PMMDataConvert/42(VINP_PWCONTINUEUSE_flg)
  PMMDataConvert/28(VPMM_DetectPWCONTINUE_flg) -> [VPMM_DetectPWCONTINUE_flg]
  [VPMM_DetectPWCONTINUE_flg] -> PMM_State_Machine/81(VPMM_DetectPWCONTINUE_flg)
  [VPMM_DetectIVIPwroffreq_flg] -> PMM_State_Machine/79(VPMM_DetectIVIPwroffreq_flg)
  [VPMM_DetectSchedChg_flg] -> PMM_State_Machine/80(VPMM_DetectSchedChg_flg)
  [VINP_EvccAplusPwrUpReq_flg] -> Data Type Conversion/1
  Data Type Conversion/1 -> VPMM_EvccAplusPwrUpReq_flg/1  "VPMM_EvccAplusPwrUpReq_flg"
  PMM_State_Machine/21(VPMM_PwrStaONTOPopReq_flg) -> VPMM_PwrStaONTOPopReq_flg/1  "VPMM_PwrStaONTOPopReq_flg"
  PMM_State_Machine/22(VPMM_IVIPwrStaONTOPopT_s) -> VPMM_IVIPwrStaONTOPopT_s/1  "VPMM_IVIPwrStaONTOPopT_s"
  PMM_State_Machine/23(VPMM_LVChrgHoldTtimer_s) -> VPMM_LVChrgHoldTtimer_s/1  "VPMM_LVChrgHoldTtimer_s"
  PMM_State_Machine/24(VPMM_LVBattChrgTimeCnt_s) -> VPMM_LVBattChrgTimeCnt_s/1  "VPMM_LVBattChrgTimeCnt_s"
  Constant36/1 -> PMM_State_Machine/82(KPMM_SilentChrgReqTO_s)
  [VINP_HoodSW_flg] -> RequirementManagementForPowerDown/13(VINP_HoodSW_flg)
  Constant37/1 -> PMM_State_Machine/83(KPMM_PwrStaONTOPop_s)
  PMM_State_Machine/26(VPMM_SilentChkAllowSleep_flg) -> VPMM_SilentChkAllowSleep_flg/1  "VPMM_SilentChkAllowSleep_flg"
  PMM_State_Machine/27(VPMM_TimerAllowSleep_flg) -> VPMM_TimerAllowSleep_flg/1  "VPMM_TimerAllowSleep_flg"
  Data Type Conversion39/1 -> VPMM_FDADC12VDetAvg_mV/1  "VPMM_FDADC12VDetAvg_mV"
  PMM_State_Machine/28(VPMM_FDADC12VDetAvg_mV) -> Gain2/1
  PMM_State_Machine/25(VPMM_PMMAllowECUSleep_flg) -> VPMM_PMMAllowECUSleep_flg/1  "VPMM_PMMAllowECUSleep_flg"
  PMM_State_Machine/29(VPMM_LVSilentChrgLv_enum) -> VPMM_LVSilentChrgLv_enum/1  "VPMM_LVSilentChrgLv_enum"
  Constant39/1 -> PMM_State_Machine/88(KPMM_LVBattOFFSlpThd_mV)
  Constant40/1 -> PMM_State_Machine/89(KPMM_OFFLVBattChkRetry_cnt)
  Constant14/1 -> PMM_State_Machine/86(KPMM_FirstLVCheckHoldT_s)
  Constant12/1 -> PMM_State_Machine/85(KPMM_FDADC12VDetAccu_s)
  Constant38/1 -> PMM_State_Machine/87(KPMM_LVBattChkWakehold_s)
  Constant6/1 -> PMM_State_Machine/84(KPMM_FDADC12VDetAccuIntval_s)
  VINP_CANMsgValidBMS2_flg/1 -> PMM_State_Machine/91(VINP_CANMsgValidBMS2_flg)
  Gain2/1 -> Data Type Conversion39/1
  PMM_State_Machine/1(VPMM_PowerUpState_enum) -> [VPMM_PowerUpState_enum]  "VPMM_PowerUpState_enum"
  PMM_State_Machine/2(VPMM_PowerDownState_enum) -> VPMM_PowerDownState_enum/1  "VPMM_PowerDownState_enum"
  PMM_State_Machine/3(VPMM_PowerUpFault_enum) -> VPMM_PowerUpFault_enum/1  "VPMM_PowerUpFault_enum"
  PMM_State_Machine/4(VPMM_PowerDownFault_enum) -> VPMM_PowerDownFault_enum/1  "VPMM_PowerDownFault_enum"
  PMM_State_Machine/5(VPMM_ActiveDischargeReq_flg) -> VPMM_ActiveDischargeReq_flg/1  "VPMM_ActiveDischargeReq_flg"
  [VPMM_SysPowerMode_enum] -> Unit Delay13/1
  [VINP_RePwrReqTbox_enum] -> RequirementManagementForPowerStateConstrain/10(VINP_RePwrReqTbox_enum)
  [VINP_RePwrReqDKCT_enum] -> RequirementManagementForPowerStateConstrain/9(VINP_RePwrReqDKCT_enum)
  [VINP_PwrReq_OTA_enum] -> RequirementManagementForPowerStateConstrain/8(VINP_PwrReq_OTA_enum)
  [VINP_PowerOffTSetDKC_enum] -> RequirementManagementForPowerStateConstrain/7(VPMM_PowerOffTSetDKC_enum)
  [VPMM_PowerOffTSet_s] -> RequirementManagementForPowerStateConstrain/6(VPMM_PowerOffTSet_s)
  [VINP_HVBPreheatPrecoolSta_enum] -> RequirementManagementForPowerStateConstrain/4(VINP_HVBPreheatPrecoolSta_enum)
  VINP_AVMOFFRecButt_flg/1 -> RequirementManagementForPowerStateConstrain/3(VINP_AVMOFFRecButt_flg)
  Unit Delay11/1 -> RequirementManagementForPowerDown/6(VPMM_PwrStaConstraint_enum)
  Unit Delay12/1 -> RequirementManagementForPowerDown/8(VPMM_TCountSta_enum)
  Unit Delay13/1 -> RequirementManagementForPowerStateConstrain/11(VPMM_PwrStaSW_enum)
  [VPMM_LVSilentChrgSta_enum] -> VPMM_LVSilentChrgSta_enum/1
  [VPMM_LVSilentChrgReq_flg] -> VPMM_LVSilentChrgReq_flg/1
  [VINP_TailgateSW_flg] -> PMM_State_Machine/97(VINP_TailgateSW_flg)
  VINP_BMSWarn6_flg/1 -> [VINP_BMSWarn6_flg]
  [VINP_BMSWarn6_flg] -> PMMDataConvert/35(VINP_BMSWarn6_flg)
  [VINP_BMSWarn6_flg] -> PMM_State_Machine/96(VINP_BMSWarn6_flg)
  [VPMM_HVPwrSta_flg] -> VPMM_HVPwrSta_flg/1
  [VPMM_AllDoorClosed_flg] -> RequirementManagementForPowerDown/14(VPMM_AllDoorClosed_flg)
  [VINP_SeatSW_flg] -> RequirementManagementForPowerDown/16(VINP_SeatSW_flg)
  [VPMM_HVPwrSta_flg] -> Unit Delay14/1
  PMMDataConvert/29(VPMM_DetectHVPwrSta_flg) -> [VPMM_DetectHVPwrSta_flg]
  [VPMM_DetectHVPwrSta_flg] -> RequirementManagementForPowerDown/15(VPMM_DetectHVPwrSta_flg)
  Constant41/1 -> RequirementManagementForPowerDown/17(KPMM_SysPwrDownDbns_s)
  Constant43/1 -> PMM_State_Machine/93(KPMM_BattUpResetSW_flg)
  Constant44/1 -> PMM_State_Machine/94(KPMM_BattUpResetTO_s)
  Constant45/1 -> PMM_State_Machine/95(KPMM_BattUpRstDlyTO_s)
  Constant42/1 -> PMM_State_Machine/92(KPMM_BattUpResetRty_cnt)
  PMM_State_Machine/32(VPMM_CtrlFrEDUINVERTER_flg) -> VPMM_CtrlFrEDUINVERTER_flg/1  "VPMM_CtrlFrEDUINVERTER_flg"
  PMM_State_Machine/33(VPMM_CtrlFrPwrStbA1P_flg) -> VPMM_CtrlFrPwrStbA1P_flg/1  "VPMM_CtrlFrPwrStbA1P_flg"
  PMM_State_Machine/34(VPMM_CtrlFrRC1_flg) -> VPMM_CtrlFrRC1_flg/1  "VPMM_CtrlFrRC1_flg"
  PMM_State_Machine/35(VPMM_HWResetSta_enum) -> VPMM_HWResetSta_enum/1  "VPMM_HWResetSta_enum"
  PMM_State_Machine/36(VPMM_HVChrgPreActionErrSta_enum) -> VPMM_HVChrgPreActionErrSta_enum/1  "VPMM_HVChrgPreActionErrSta_enum"
  PMM_State_Machine/30(VPMM_CtrlDrPwrStbA2_flg) -> VPMM_CtrlDrPwrStbA2_flg/1  "VPMM_CtrlDrPwrStbA2_flg"
  PMM_State_Machine/31(VPMM_CtrlFrBMSCCUCIR_flg) -> VPMM_CtrlFrBMSCCUCIR_flg/1  "VPMM_CtrlFrBMSCCUCIR_flg"
  PMMDataConvert/30(VPMM_MCUReady4Pre_flg) -> VPMM_MCUReady4Pre_flg/1
  [VPMM_SafetyChkMLv_flg] -> VPMM_SafetyChkMLv_flg/1
  [VPMM_SafetyChkHLv_flg] -> VPMM_SafetyChkHLv_flg/1
  [VPMM_MCUReady_flg] -> VPMM_MCUReady_flg/1
  Unit Delay14/1 -> PMMDataConvert/43(VPMM_HVPwrSta_flg)
  [VPMM_BrkPedalPressed_flg] -> RequirementManagementForPowerDown/18(VPMM_BrkPedalPressed_flg)
  [VPMM_PwrStaTOSta_enum] -> VPMM_PwrStaTOSta_enum/1
  Constant46/1 -> PMM_State_Machine/98(KPMM_HoodOffChkFailtime_s)
  Constant28/1 -> RequirementManagementForPowerDown/20(KPMM_HVBattSOCPwrDwnThd_pct)
  [VINP_EvccAplusPwrUpReq_flg] -> RequirementManagementForPowerDown/19(VINP_EvccAplusPwrUpReq_flg)
  [VPMM_PowerSta_enum] -> DCDC output volt setpoint judgment/2(VPMM_PowerSta_enum)
  [VPMM_HVPwrSta_flg] -> DCDC output volt setpoint judgment/3(VPMM_HVPwrSta_flg)
  [VPMM_LVSilentChrgReq_flg] -> DCDC output volt setpoint judgment/4(VPMM_LVSilentChrgReq_flg)
  [VPMM_LVSilentChrgReqStd_flg] -> DCDC output volt setpoint judgment/5(VPMM_LVSilentChrgReqStd_flg)
  DCDC output volt setpoint judgment/1(VPMM_DCDCVoltSetpoint_V) -> VPMM_DCDCVoltSetpoint_V/1  "VPMM_DCDCVoltSetpoint_V"
  PMM_State_Machine/7(VPMM_DCDCVoltSetpointPU_V) -> [VPMM_DCDCVoltSetpointPU_V]  "VPMM_DCDCVoltSetpointPU_V"
  [VPMM_DCDCVoltSetpointPU_V] -> DCDC output volt setpoint judgment/1(VPMM_DCDCVoltSetpointPU_V)
  Constant27/1 -> PMM_State_Machine/99(KPMM_HVSOCWarnThd_pct)
  VINP_OFFACMODE_enum/1 -> [VINP_OFFACMODE_enum]
  [VINP_OFFACMODE_enum] -> RequirementManagementForPowerStateConstrain/5(VINP_OFFACMODE_enum)
  [VINP_OFFACMODE_enum] -> PMM_State_Machine/100(VINP_OFFACMODE_enum)
  VINP_V2LSta_enum/1 -> PMM_State_Machine/101(VINP_V2LSta_enum)
  VINP_PsDoorSW_flg/1 -> [VINP_PsDoorSW_flg]
  VINP_RRDoorSW_flg/1 -> [VINP_RRDoorSW_flg]
  VINP_RLDoorSW_flg/1 -> [VINP_RLDoorSW_flg]
  [VINP_PsDoorSW_flg] -> PMMDataConvert/4(VINP_PsDoorSW_flg)
  [VINP_RRDoorSW_flg] -> PMMDataConvert/5(VINP_RRDoorSW_flg)
  [VINP_RLDoorSW_flg] -> PMMDataConvert/6(VINP_RLDoorSW_flg)
  [VINP_PsDoorSW_flg] -> PMM_State_Machine/102(VINP_PsDoorSW_flg)
  [VINP_RRDoorSW_flg] -> PMM_State_Machine/103(VINP_RRDoorSW_flg)
  [VINP_RLDoorSW_flg] -> PMM_State_Machine/104(VINP_RLDoorSW_flg)
  [VINP_RLDoorSW_flg] -> Detect Increase2/1
  [VINP_RRDoorSW_flg] -> Detect Increase1/1
  [VINP_PsDoorSW_flg] -> Detect Increase/1
  [VINP_SeatSW_flg] -> Detect Decrease/1
  Detect Decrease/1 -> PMM_State_Machine/108(VPMM_DetectSeatEmpty_flg)  "VPMM_DetectSeatEmpty_flg"
  Detect Increase/1 -> PMM_State_Machine/105(VPMM_DetectPsDoorOpened_flg)  "VPMM_DetectPsDoorOpened_flg"
  Detect Increase2/1 -> PMM_State_Machine/106(VPMM_DetectRLDoorOpened_flg)  "VPMM_DetectRLDoorOpened_flg"
  Detect Increase1/1 -> PMM_State_Machine/107(VPMM_DetectRRDoorOpened_flg)  "VPMM_DetectRRDoorOpened_flg"
  VINP_LVBattDet12V_V/1 -> Data Type Conversion1/1
  Data Type Conversion1/1 -> [VINP_LVBattDet12V_V], PMM_State_Machine/24(VINP_LVBattDet12V_V)
  PMM_State_Machine/37(VPMM_PMMAllowNMSleep_flg) -> VPMM_PMMAllowNMSleep_flg/1  "VPMM_PMMAllowNMSleep_flg"
  Gain1/1 -> Data Type Conversion2/1
  [VINP_LVBattDet12V_V] -> Gain1/1
  Data Type Conversion2/1 -> PMM_State_Machine/90(VINP_LvBattVolt_mV)
  [VINP_PwrReq_OTA_enum] -> OTA power state constrain/2(VINP_PwrReq_OTA_enum)
  [VPMM_PowerSta_enum] -> OTA power state constrain/3(VPMM_PowerSta_enum)
  [task_time_s] -> OTA power state constrain/1(task_time_s)
  OTA power state constrain/1(VPMM_OTAPwrReqOFFChkSta_enum) -> [VPMM_OTAPwrReqOFFChkSta_enum]  "VPMM_OTAPwrReqOFFChkSta_enum"
  OTA power state constrain/2(VPMM_OTAPwrReqStdChkSta_enum) -> [VPMM_OTAPwrReqStdChkSta_enum]  "VPMM_OTAPwrReqStdChkSta_enum"
  [VPMM_OTAPwrReqOFFChkSta_enum] -> Unit Delay15/1
  [VPMM_OTAPwrReqStdChkSta_enum] -> Unit Delay16/1
  Unit Delay15/1 -> PMM_State_Machine/109(VPMM_OTAPwrReqOFFChkSta_enum)
  Unit Delay16/1 -> PMM_State_Machine/110(VPMM_OTAPwrReqStdChkSta_enum)
  [VPMM_OTAPwrReqOFFChkSta_enum] -> Unit Delay17/1
  [VPMM_OTAPwrReqStdChkSta_enum] -> Unit Delay18/1
  [VINP_PwrReq_OTA_enum] -> Data Type Conversion3/1
  Data Type Conversion3/1 -> VPMM_PwrReq_OTA_enum/1  "VPMM_PwrReq_OTA_enum"
  [VPMM_OTAPwrReqStdChkSta_enum] -> VPMM_OTAPwrReqStdChkSta_enum/1
  [VPMM_OTAPwrReqOFFChkSta_enum] -> VPMM_OTAPwrReqOFFChkSta_enum/1
  [VPMM_Sched_ChgTOSta_enum] -> VPMM_Sched_ChgTOSta_enum/1
  Unit Delay17/1 -> RequirementManagementForPowerUp/26(VPMM_OTAPwrReqOFFChkSta_enum)
  Unit Delay18/1 -> RequirementManagementForPowerUp/27(VPMM_OTAPwrReqStdChkSta_enum)
  Constant47/1 -> RequirementManagementForPowerUp/28(KPMM_HVBattSOCPwrDwnThd_pct)
  [VPMM_OTAPwrReqOFFChkSta_enum] -> Unit Delay19/1
  Unit Delay19/1 -> RequirementManagementForPowerDown/21(VPMM_OTAPwrReqOFFChkSta_enum)
  Constant35/1 -> RequirementManagementForPowerDown/12(KPMM_HVSOCWarnTime_s)
  [VPMM_MCUDCBusMaxVolt_V] -> VPMM_MCUDCBusMaxVolt_V/1  "VPMM_MCUDCBusMaxVolt_V"
  Data Type Conversion4/1 -> [task_time_s]

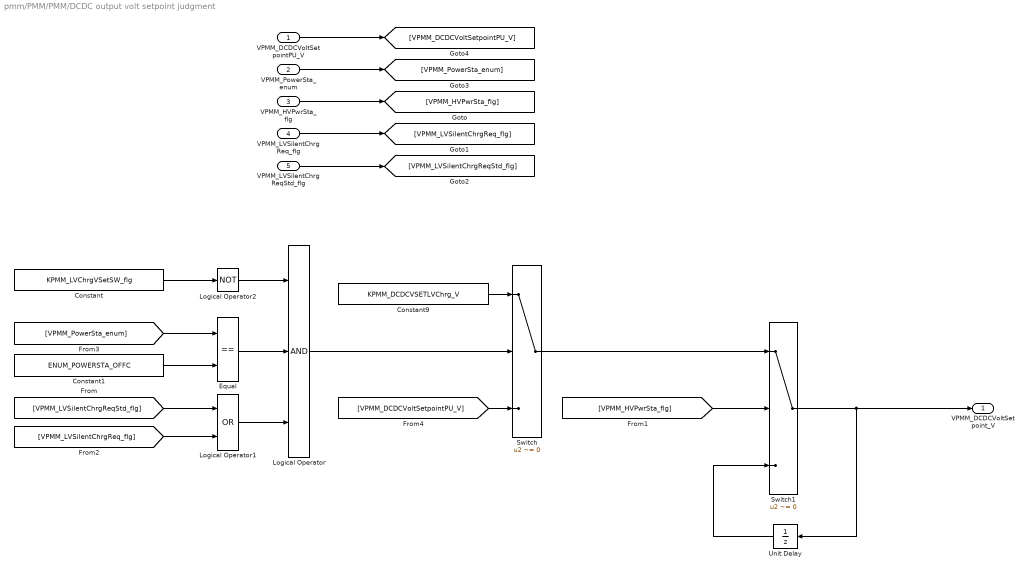
== system pmm/PMM/PMM/DCDC output volt setpoint judgment ==
  VPMM_DCDCVoltSetpointPU_V : Inport
  VPMM_PowerSta_enum : Inport  Port=2
  VPMM_HVPwrSta_flg : Inport  Port=3
  VPMM_LVSilentChrgReq_flg : Inport  Port=4
  VPMM_LVSilentChrgReqStd_flg : Inport  Port=5
  Constant : Constant  Value=KPMM_LVChrgVSetSW_flg
  Constant1 : Constant  Value=ENUM_POWERSTA_OFFC
  Constant9 : Constant  Value=KPMM_DCDCVSETLVChrg_V
  Equal : RelationalOperator  Operator===  OutDataTypeStr=boolean  RndMeth=Simplest
  Logical Operator : Logic  Inputs=3  AllPortsSameDT=off  OutDataTypeStr=boolean
  Logical Operator1 : Logic  Operator=OR  AllPortsSameDT=off  OutDataTypeStr=boolean
  Logical Operator2 : Logic  Operator=NOT  AllPortsSameDT=off  OutDataTypeStr=boolean
  Switch : Switch  Criteria=u2 ~= 0
  Switch1 : Switch  Criteria=u2 ~= 0
  Unit Delay : UnitDelay  SampleTime=-1  HasFrameUpgradeWarning=on
  VPMM_DCDCVoltSetpoint_V : Outport
  wires:
  Switch1/1 -> VPMM_DCDCVoltSetpoint_V/1, Unit Delay/1
  VPMM_PowerSta_enum/1 -> [VPMM_PowerSta_enum]
  VPMM_HVPwrSta_flg/1 -> [VPMM_HVPwrSta_flg]
  VPMM_LVSilentChrgReq_flg/1 -> [VPMM_LVSilentChrgReq_flg]
  VPMM_LVSilentChrgReqStd_flg/1 -> [VPMM_LVSilentChrgReqStd_flg]
  VPMM_DCDCVoltSetpointPU_V/1 -> [VPMM_DCDCVoltSetpointPU_V]
  Constant9/1 -> Switch/1
  Equal/1 -> Logical Operator/2
  Unit Delay/1 -> Switch1/3
  Switch/1 -> Switch1/1
  Logical Operator/1 -> Switch/2
  [VPMM_LVSilentChrgReq_flg] -> Logical Operator1/2
  [VPMM_LVSilentChrgReqStd_flg] -> Logical Operator1/1
  Logical Operator1/1 -> Logical Operator/3
  [VPMM_HVPwrSta_flg] -> Switch1/2
  Constant1/1 -> Equal/2
  [VPMM_PowerSta_enum] -> Equal/1
  [VPMM_DCDCVoltSetpointPU_V] -> Switch/3
  Logical Operator2/1 -> Logical Operator/1
  Constant/1 -> Logical Operator2/1

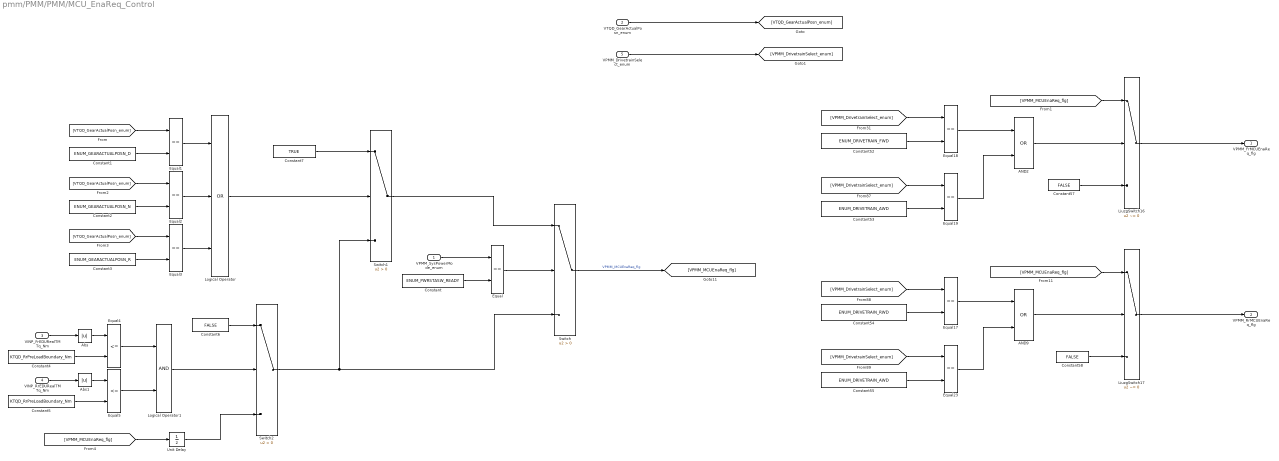
== system pmm/PMM/PMM/MCU_EnaReq_Control ==
  VPMM_SysPowerMode_enum : Inport
  VTQD_GearActualPosn_enum : Inport  Port=2
  VINP_FrEDURealTMTq_Nm : Inport  Port=3
  VINP_RrEDURealTMTq_Nm : Inport  Port=4
  VPMM_DrivetrainSelect_enum : Inport  Port=5
  AND2 : Logic  Operator=OR  AllPortsSameDT=off  OutDataTypeStr=boolean
  AND9 : Logic  Operator=OR  AllPortsSameDT=off  OutDataTypeStr=boolean
  Abs : Abs
  Abs1 : Abs
  Constant : Constant  Value=ENUM_PWRSTASW_READY
  Constant1 : Constant  Value=ENUM_GEARACTUALPOSN_D
  Constant2 : Constant  Value=ENUM_GEARACTUALPOSN_N
  Constant3 : Constant  Value=ENUM_GEARACTUALPOSN_R
  Constant4 : Constant  Value=KTQD_RrPreLoadBoundary_Nm
  Constant5 : Constant  Value=KTQD_RrPreLoadBoundary_Nm
  Constant52 : Constant  Value=ENUM_DRIVETRAIN_FWD
  Constant53 : Constant  Value=ENUM_DRIVETRAIN_AWD
  Constant54 : Constant  Value=ENUM_DRIVETRAIN_RWD
  Constant55 : Constant  Value=ENUM_DRIVETRAIN_AWD
  Constant57 : Constant  Value=FALSE
  Constant58 : Constant  Value=FALSE
  Constant6 : Constant  Value=FALSE
  Constant7 : Constant  Value=TRUE
  Equal{,1..3,17..19,23} (8 alike) : RelationalOperator  Operator===  OutDataTypeStr=boolean  RndMeth=Simplest
  Equal4 : RelationalOperator  Operator=<=  OutDataTypeStr=boolean  RndMeth=Simplest
  Equal5 : RelationalOperator  Operator=<=  OutDataTypeStr=boolean  RndMeth=Simplest
  LiuzgSwitch16 : Switch  Criteria=u2 ~= 0
      settings: AttributesFormatString=<%<Criteria>>
  LiuzgSwitch17 : Switch  Criteria=u2 ~= 0
      settings: AttributesFormatString=<%<Criteria>>
  Logical Operator : Logic  Operator=OR  Inputs=3  AllPortsSameDT=off  OutDataTypeStr=boolean
  Logical Operator1 : Logic  AllPortsSameDT=off  OutDataTypeStr=boolean
  Switch : Switch  Criteria=u2 > Threshold
  Switch1 : Switch  Criteria=u2 > Threshold
  Switch2 : Switch  Criteria=u2 > Threshold
  Unit Delay : UnitDelay  SampleTime=-1  HasFrameUpgradeWarning=on
  VPMM_FrMCUEnaReq_flg : Outport
  VPMM_RrMCUEnaReq_flg : Outport  Port=2
  wires:
  VPMM_DrivetrainSelect_enum/1 -> [VPMM_DrivetrainSelect_enum]
  LiuzgSwitch17/1 -> VPMM_RrMCUEnaReq_flg/1
  Constant57/1 -> LiuzgSwitch16/3
  [VPMM_DrivetrainSelect_enum] -> Equal19/1
  Constant55/1 -> Equal23/2
  Constant58/1 -> LiuzgSwitch17/3
  Constant54/1 -> Equal17/2
  Constant53/1 -> Equal19/2
  Equal19/1 -> AND2/2
  [VPMM_DrivetrainSelect_enum] -> Equal17/1
  [VPMM_MCUEnaReq_flg] -> LiuzgSwitch16/1
  [VPMM_MCUEnaReq_flg] -> LiuzgSwitch17/1
  AND2/1 -> LiuzgSwitch16/2
  [VPMM_DrivetrainSelect_enum] -> Equal23/1
  Equal17/1 -> AND9/1
  Constant52/1 -> Equal18/2
  [VPMM_DrivetrainSelect_enum] -> Equal18/1
  Equal18/1 -> AND2/1
  LiuzgSwitch16/1 -> VPMM_FrMCUEnaReq_flg/1
  AND9/1 -> LiuzgSwitch17/2
  Equal23/1 -> AND9/2
  VPMM_SysPowerMode_enum/1 -> Equal/1
  Constant/1 -> Equal/2
  Equal/1 -> Switch/2
  Switch1/1 -> Switch/1
  Switch/1 -> [VPMM_MCUEnaReq_flg]  "VPMM_MCUEnaReq_flg"
  VTQD_GearActualPosn_enum/1 -> [VTQD_GearActualPosn_enum]
  [VTQD_GearActualPosn_enum] -> Equal1/1
  [VTQD_GearActualPosn_enum] -> Equal2/1
  [VTQD_GearActualPosn_enum] -> Equal3/1
  Constant3/1 -> Equal3/2
  Constant2/1 -> Equal2/2
  Constant1/1 -> Equal1/2
  Equal3/1 -> Logical Operator/3
  Equal2/1 -> Logical Operator/2
  Equal1/1 -> Logical Operator/1
  Logical Operator/1 -> Switch1/2
  Switch2/1 -> Switch1/3, Switch/3
  Equal4/1 -> Logical Operator1/1
  Equal5/1 -> Logical Operator1/2
  Logical Operator1/1 -> Switch2/2
  VINP_FrEDURealTMTq_Nm/1 -> Abs/1
  VINP_RrEDURealTMTq_Nm/1 -> Abs1/1
  Constant4/1 -> Equal4/2
  Constant5/1 -> Equal5/2
  [VPMM_MCUEnaReq_flg] -> Unit Delay/1
  Unit Delay/1 -> Switch2/3
  Constant6/1 -> Switch2/1
  Constant7/1 -> Switch1/1
  Abs/1 -> Equal4/1
  Abs1/1 -> Equal5/1
